simulink model "aeroelastic_feedback"  (R2024b)
settings: Solver=ode15s  StartTime=0.0  StopTime=1  RelTol=1e-3  AbsTol=1e-10
undefined symbols (not defined in the file): AEROELASTIC, AOA, areas, Brom, chord, coeffs, Crom, Kode, nIn, nStations, rho, tw, tw_sub, Vinf
libraries: simulink_extras x1
settings Model: Creator=jclinton  LastModifiedBy=jclinton
settings DataIOCC: SaveFormat=Array

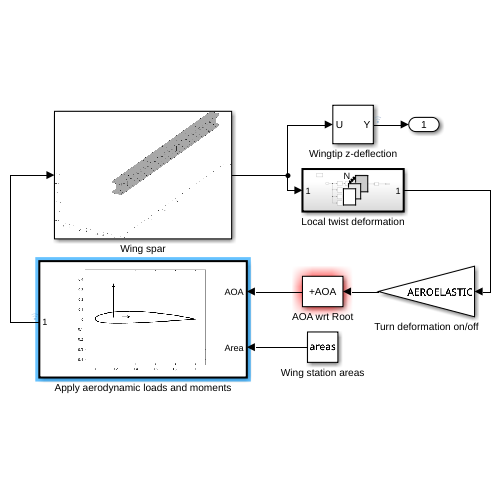
[thumbnail: Simulink's stored preview of the top-level diagram]
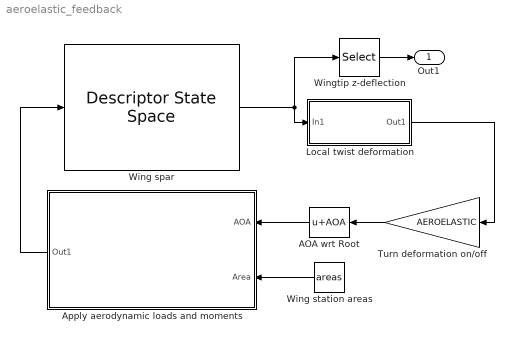
== system aeroelastic_feedback ==
  AOA wrt Root : Bias  Bias=AOA  SaturateOnIntegerOverflow=off
  Apply aerodynamic loads and moments : Subsystem  TreatAsAtomicUnit=on
      mask Display: image('airfoilLD.png', [0,0,0,0,100,100]);
  Local twist deformation : Subsystem  TreatAsAtomicUnit=on
  Turn deformation on/off : Gain  Gain=AEROELASTIC
  Wing spar : DescriptorStateSpace  E=Mode  A=-Kode  B=Brom  C=Crom  D=zeros(size(Crom,1),nIn)  InitialCondition=0  DirectFeedthrough=False
      mask Display: image('beam.png');
  Wing station areas : Constant  Value=areas
  Wingtip z-deflection : Selector  InputPortWidth=4*nStations  IndexOptions=Index vector (dialog)  Indices=4*nStations  OutputSizes=1
  Out1 : Outport
  wires:
  Local twist deformation/1(Out1) -> Turn deformation on/off/1
  Apply aerodynamic loads and moments/1(Out1) -> Wing spar/1
  AOA wrt Root/1 -> Apply aerodynamic loads and moments/1(AOA)
  Turn deformation on/off/1 -> AOA wrt Root/1
  Wing station areas/1 -> Apply aerodynamic loads and moments/2(Area)
  Wingtip z-deflection/1 -> Out1/1
  Wing spar/1 -> Wingtip z-deflection/1, Local twist deformation/1(In1)

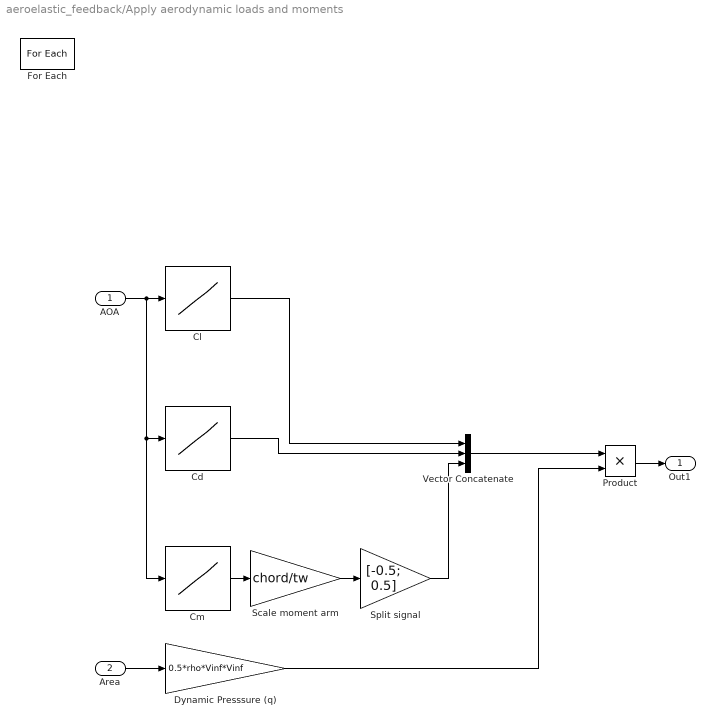
== system aeroelastic_feedback/Apply aerodynamic loads and moments ==
  AOA : Inport  Partition=on  PartitionDimension=1  PartitionWidth=1  PartitionOffset=0
  Area : Inport  Port=2  Partition=on  PartitionDimension=1  PartitionWidth=1  PartitionOffset=0
  Cd : Lookup_n-D  NumberOfTableDimensions=1  BreakpointsForDimension1=coeffs(:,1)  Table=coeffs(:,3)  InternalRulePriority=Speed  RndMeth=Simplest
  Cl : Lookup_n-D  NumberOfTableDimensions=1  BreakpointsForDimension1=coeffs(:,1)  Table=coeffs(:,2)  InternalRulePriority=Speed  RndMeth=Simplest
  Cm : Lookup_n-D  NumberOfTableDimensions=1  BreakpointsForDimension1=coeffs(:,1)  Table=coeffs(:,4)  InternalRulePriority=Speed  RndMeth=Simplest
  Dynamic Presssure (q) : Gain  Gain=0.5*rho*Vinf*Vinf
  For Each : ForEach  DisableCoverage=on
  Product : Product
  Scale moment arm : Gain  Gain=chord/tw
  Split signal : Gain  Gain=[-0.5; 0.5]
  Vector Concatenate : Concatenate  NumInputs=3
  Out1 : Outport  ConcatenationDimension=1
  wires:
  AOA/1 -> Cm/1, Cd/1, Cl/1
  Area/1 -> Dynamic Presssure (q)/1
  Product/1 -> Out1/1
  Cd/1 -> Vector Concatenate/2
  Cl/1 -> Vector Concatenate/1
  Dynamic Presssure (q)/1 -> Product/2
  Vector Concatenate/1 -> Product/1
  Cm/1 -> Scale moment arm/1
  Scale moment arm/1 -> Split signal/1
  Split signal/1 -> Vector Concatenate/3

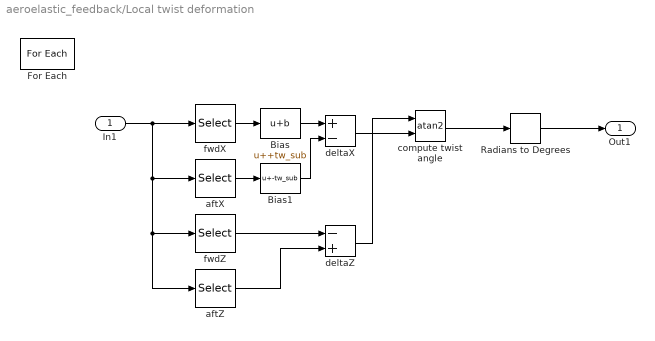
== system aeroelastic_feedback/Local twist deformation ==
  In1 : Inport  Partition=on  PartitionDimension=1  PartitionWidth=4  PartitionOffset=0
  Bias : Bias  Bias=+tw_sub  SaturateOnIntegerOverflow=off
  Bias1 : Bias  Bias=-tw_sub  SaturateOnIntegerOverflow=off
  For Each : ForEach  DisableCoverage=on
  Radians to Degrees : simulink_extras/Transformations/Radians to Degrees
  aftX : Selector  InputPortWidth=4  IndexOptions=Index vector (dialog)  Indices=2  OutputSizes=1
  aftZ : Selector  InputPortWidth=4  IndexOptions=Index vector (dialog)  Indices=4  OutputSizes=1
  compute twist angle : Trigonometry  Operator=atan2
  deltaX : Sum  Inputs=+-
  deltaZ : Sum  Inputs=-+
  fwdX : Selector  InputPortWidth=4  IndexOptions=Index vector (dialog)  Indices=1  OutputSizes=1
  fwdZ : Selector  InputPortWidth=4  IndexOptions=Index vector (dialog)  Indices=3  OutputSizes=1
  Out1 : Outport  ConcatenationDimension=1
  wires:
  fwdX/1 -> Bias/1
  aftX/1 -> Bias1/1
  Bias/1 -> deltaX/1
  Bias1/1 -> deltaX/2
  fwdZ/1 -> deltaZ/1
  aftZ/1 -> deltaZ/2
  deltaX/1 -> compute twist angle/2
  deltaZ/1 -> compute twist angle/1
  Radians to Degrees/1 -> Out1/1
  compute twist angle/1 -> Radians to Degrees/1
  In1/1 -> aftZ/1, fwdZ/1, aftX/1, fwdX/1
